simulink model "String3_Diode_P"  (R2023b)
settings: Solver=VariableStepAuto  StartTime=0.0  StopTime=10.0  RelTol=1e-3
undefined symbols (not defined in the file or in its folder): Slope_Vdc_string3
libraries: SolarCellLibrary x20, spsCurrentMeasurementLib x1, spsControlledVoltageSourceLib x1, simulink x1, spsVoltageMeasurementLib x1
settings Model: Creator=kevin  LastModifiedBy=kevin

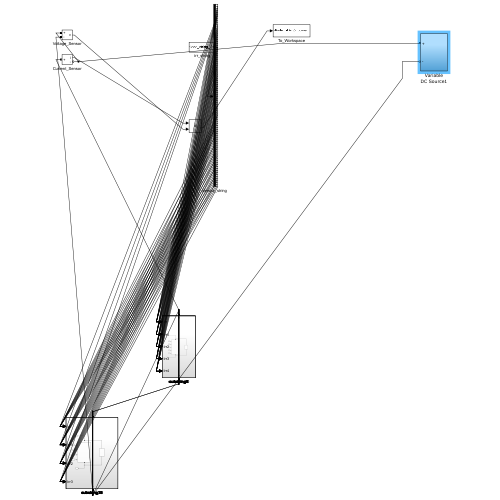
[thumbnail: Simulink's stored preview of the top-level diagram]
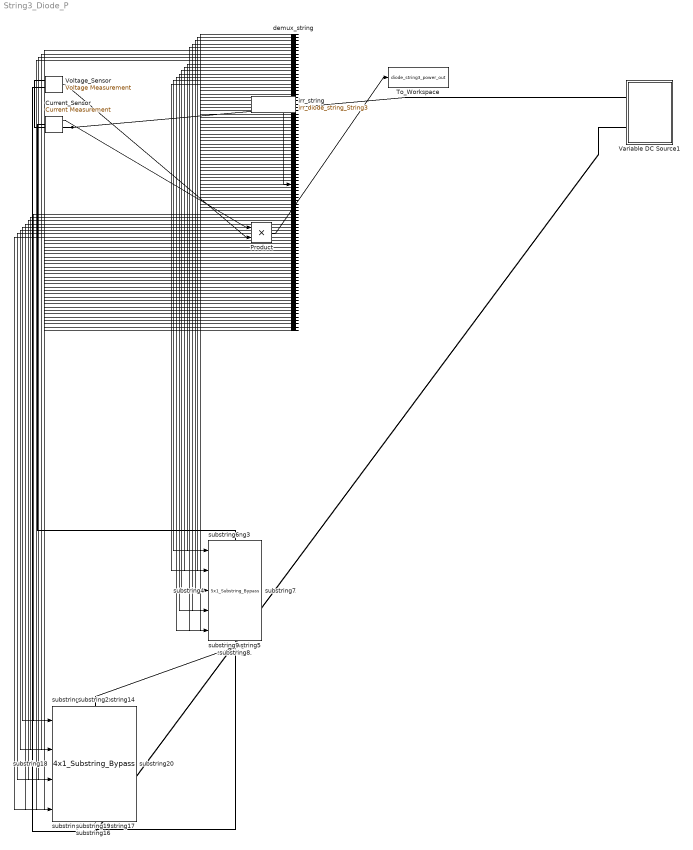
== system String3_Diode_P ==
  Current_Sensor : spsCurrentMeasurementLib/Current Measurement  PhasorSimulation=off  OutputType=Complex  PSBequivalent=0
  Product : Product
  To_Workspace : ToWorkspace  VariableName=diode_string3_power_out  SaveFormat=Timeseries  SampleTime=-1
  Variable DC Source1 : Subsystem
  Voltage_Sensor : spsVoltageMeasurementLib/Voltage Measurement  PhasorSimulation=off  OutputType=Complex  PSBequivalent=0
  demux_string : Demux  Outputs=90
  irr_string : FromWorkspace  VariableName=irr_diode_string_String3
  substring{1,3..11} (10 alike) : SolarCellLibrary/5x1_Substring_Bypass  SystemSampleTime=-1  VariantActivationTime=update diagram  AllowFlexibleInterface=on  Latency=0  AutoFrameSizeCalculation=off
      settings: PortSchema="{\"entries\":[{\"content\":{\"sides\":[{\"content\":{\"connectorIds\":[\"In1\",\"In2\",\"In3\",\"In4\",\"In5\"]},\"type\":\"ConnectorPlacement.EquallySpacedRectSide\",\"uuid\":\"51ad4193-b089-4581-a8f5-cdd81cf51d92\"},{\"content\":{\"side\":\"RIGHT\"},\"type\":\"ConnectorPlacement.EquallySpacedRectSide\",\"uuid\":\"beefcb7b-5e98-41ac-8640-136b2bf4d9bd\"},{\"content\":{\"connectorIds\":[\"LConn1\"],\"side\":\"TOP\"},\"type\":\"ConnectorPlacement.EquallySpacedRectSide\",\"uuid\":\"09275b5d-5163-48bd-952c-35e4981d85a7\"},{\"content\":{\"connectorIds\":[\"RConn1\"],\"side\":\"BOTTOM\"},\"type\":\"ConnectorPlacement.EquallySpacedRectSide\",\"uuid\":\"1e8d88ef-9c7a-4e42-9471-00569e7c3c03\"}]},\"type\":\"ConnectorPlacement.EquallySpacedConnector\",\"uuid\":\"d217ca46-39f3-4298-b827-e58aec46a1ce\"}],\"packageUris\":[\"http://schema.mathworks.com/mf0/Connector/R2020b\"],\"version\":\"1.0\"}"
  substring{2,12..20} (10 alike) : SolarCellLibrary/4x1_Substring_Bypass  SystemSampleTime=-1  VariantActivationTime=update diagram  AllowFlexibleInterface=on  Latency=0  AutoFrameSizeCalculation=off
      settings: PortSchema="{\"entries\":[{\"content\":{\"sides\":[{\"content\":{\"connectorIds\":[\"In1\",\"In2\",\"In3\",\"In4\"]},\"type\":\"ConnectorPlacement.EquallySpacedRectSide\",\"uuid\":\"0ad94482-327f-42a8-a753-929b8c21c598\"},{\"content\":{\"side\":\"RIGHT\"},\"type\":\"ConnectorPlacement.EquallySpacedRectSide\",\"uuid\":\"447f9d08-5865-4684-a5c5-74ffbb93afc8\"},{\"content\":{\"connectorIds\":[\"LConn1\"],\"side\":\"TOP\"},\"type\":\"ConnectorPlacement.EquallySpacedRectSide\",\"uuid\":\"4f0b0805-593f-452f-8bf0-062e33ae5583\"},{\"content\":{\"connectorIds\":[\"RConn1\"],\"side\":\"BOTTOM\"},\"type\":\"ConnectorPlacement.EquallySpacedRectSide\",\"uuid\":\"b069b9dc-d744-4b07-9d86-0222f837bdcc\"}]},\"type\":\"ConnectorPlacement.EquallySpacedConnector\",\"uuid\":\"0517c35b-d064-4567-8e0e-3ac38b35b549\"}],\"packageUris\":[\"http://schema.mathworks.com/mf0/Connector/R2020b\"],\"version\":\"1.0\"}"
  wires:
  irr_string/1 -> demux_string/1
  demux_string/1 -> substring1/1
  demux_string/2 -> substring1/2
  demux_string/3 -> substring1/3
  demux_string/4 -> substring1/4
  demux_string/5 -> substring1/5
  demux_string/6 -> substring2/1
  demux_string/7 -> substring2/2
  demux_string/8 -> substring2/3
  demux_string/9 -> substring2/4
  demux_string/10 -> substring3/1
  demux_string/11 -> substring3/2
  demux_string/12 -> substring3/3
  demux_string/13 -> substring3/4
  demux_string/14 -> substring3/5
  demux_string/15 -> substring4/1
  demux_string/16 -> substring4/2
  demux_string/17 -> substring4/3
  demux_string/18 -> substring4/4
  demux_string/19 -> substring4/5
  demux_string/20 -> substring5/1
  demux_string/21 -> substring5/2
  demux_string/22 -> substring5/3
  demux_string/23 -> substring5/4
  demux_string/24 -> substring5/5
  demux_string/25 -> substring6/1
  demux_string/26 -> substring6/2
  demux_string/27 -> substring6/3
  demux_string/28 -> substring6/4
  demux_string/29 -> substring6/5
  demux_string/30 -> substring7/1
  demux_string/31 -> substring7/2
  demux_string/32 -> substring7/3
  demux_string/33 -> substring7/4
  demux_string/34 -> substring7/5
  demux_string/35 -> substring8/1
  demux_string/36 -> substring8/2
  demux_string/37 -> substring8/3
  demux_string/38 -> substring8/4
  demux_string/39 -> substring8/5
  demux_string/40 -> substring9/1
  demux_string/41 -> substring9/2
  demux_string/42 -> substring9/3
  demux_string/43 -> substring9/4
  demux_string/44 -> substring9/5
  demux_string/45 -> substring10/1
  demux_string/46 -> substring10/2
  demux_string/47 -> substring10/3
  demux_string/48 -> substring10/4
  demux_string/49 -> substring10/5
  demux_string/50 -> substring11/1
  demux_string/51 -> substring11/2
  demux_string/52 -> substring11/3
  demux_string/53 -> substring11/4
  demux_string/54 -> substring11/5
  demux_string/55 -> substring12/1
  demux_string/56 -> substring12/2
  demux_string/57 -> substring12/3
  demux_string/58 -> substring12/4
  demux_string/59 -> substring13/1
  demux_string/60 -> substring13/2
  demux_string/61 -> substring13/3
  demux_string/62 -> substring13/4
  demux_string/63 -> substring14/1
  demux_string/64 -> substring14/2
  demux_string/65 -> substring14/3
  demux_string/66 -> substring14/4
  demux_string/67 -> substring15/1
  demux_string/68 -> substring15/2
  demux_string/69 -> substring15/3
  demux_string/70 -> substring15/4
  demux_string/71 -> substring16/1
  demux_string/72 -> substring16/2
  demux_string/73 -> substring16/3
  demux_string/74 -> substring16/4
  demux_string/75 -> substring17/1
  demux_string/76 -> substring17/2
  demux_string/77 -> substring17/3
  demux_string/78 -> substring17/4
  demux_string/79 -> substring18/1
  demux_string/80 -> substring18/2
  demux_string/81 -> substring18/3
  demux_string/82 -> substring18/4
  demux_string/83 -> substring19/1
  demux_string/84 -> substring19/2
  demux_string/85 -> substring19/3
  demux_string/86 -> substring19/4
  demux_string/87 -> substring20/1
  demux_string/88 -> substring20/2
  demux_string/89 -> substring20/3
  demux_string/90 -> substring20/4
  Current_Sensor/1 -> Product/1
  Voltage_Sensor/1 -> Product/2
  Product/1 -> To_Workspace/1
  connections:
  substring2/LConn1 -- substring1/RConn1
  substring3/LConn1 -- substring2/RConn1
  substring4/LConn1 -- substring3/RConn1
  substring5/LConn1 -- substring4/RConn1
  substring6/LConn1 -- substring5/RConn1
  substring7/LConn1 -- substring6/RConn1
  substring8/LConn1 -- substring7/RConn1
  substring9/LConn1 -- substring8/RConn1
  substring10/LConn1 -- substring9/RConn1
  substring11/LConn1 -- substring10/RConn1
  substring12/LConn1 -- substring11/RConn1
  substring13/LConn1 -- substring12/RConn1
  substring14/LConn1 -- substring13/RConn1
  substring15/LConn1 -- substring14/RConn1
  substring16/LConn1 -- substring15/RConn1
  substring17/LConn1 -- substring16/RConn1
  substring18/LConn1 -- substring17/RConn1
  substring19/LConn1 -- substring18/RConn1
  substring20/LConn1 -- substring19/RConn1
  substring1/LConn1 -- Current_Sensor/LConn1
  Current_Sensor/RConn1 -- Variable DC Source1/LConn1 -- Voltage_Sensor/LConn1
  substring20/RConn1 -- Variable DC Source1/LConn2 -- Voltage_Sensor/LConn2

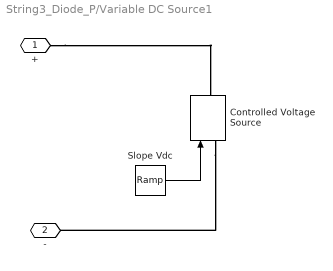
== system String3_Diode_P/Variable DC Source1 ==
  Controlled Voltage Source : spsControlledVoltageSourceLib/Controlled Voltage Source  Initialize=on  Source_Type=DC  Amplitude=0  Phase=0  Frequency=0  Measurements=None
  Slope Vdc : simulink/Sources/Ramp  slope=Slope_Vdc_string3  start=0  InitialOutput=0
  + : PMIOPort  Side=Left
  - : PMIOPort  Port=2  Side=Left
  wires:
  Slope Vdc/1 -> Controlled Voltage Source/1
  connections:
  Controlled Voltage Source/LConn1 -- -/RConn1
  +/RConn1 -- Controlled Voltage Source/RConn1
